simulink model "mypid2"  (R2024b)
settings: Solver=ode4  StartTime=0.0  StopTime=60  FixedStep=1e-3  RelTol=1e-3
StopFcn:
  | data = out.simout;
  | 
  | figure
  | subplot(2,1,1)
  | hold on
  | plot(data(:,1), data(:,2), 'LineWidth', 2, 'Color', 'r')
  | plot(data(:,1), data(:,3), 'LineWidth', 8, 'Color', 'b')
  | plot(data(:,1), data(:,4), 'LineWidth', 2, 'Color', 'k')
  | 
  | legend('Set vale', 'By MATLAB Simulink', 'By our discretization')
  | xlabel('Time (seconds)')
  | ylabel('Output')
  | 
  | subplot(2,1,2)
  | plot(data(:,1),abs(data(:,3)-data(:,4)), 'LineWidth', 2, 'Color', 'r')
  | xlabel('Time (seconds)')
  | ylabel('Absolute differences')
libraries: slpidlib x1, SignalEditorBlockLib x1
settings Model: Creator=auralius  LastModifiedBy=auralius

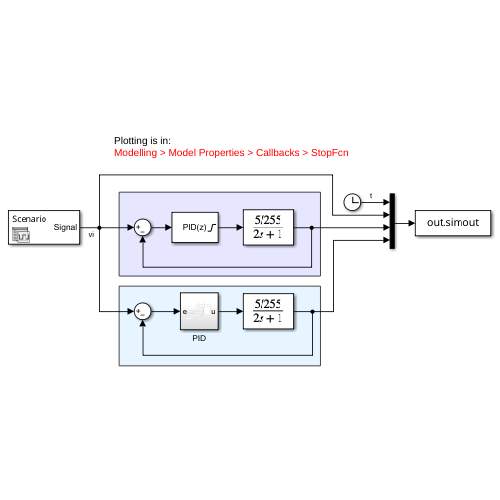
[thumbnail: Simulink's stored preview of the top-level diagram]
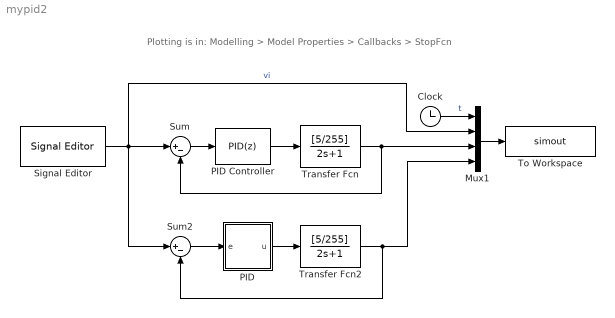
== system mypid2 ==
  note: Plotting is in:
      | Modelling > Model Properties > Callbacks > StopFcn
  Clock : Clock
  Mux1 : Mux
  PID : Subsystem
  PID Controller : slpidlib/PID Controller  Controller=PID  Form=Parallel  TimeDomain=Discrete-time  UseExternalTs=off  SampleTime=-1  IntegratorMethod=Trapezoidal  FilterMethod=Trapezoidal  ControllerParametersSource=internal  P=100  I=100  UseKiTs=off  D=10  UseExternalDerivativeSource=off  N=100  UseFilter=on  TunerSelectOption=Transfer Function Based (PID Tuner App)  ZeroCross=off  InitialConditionSource=internal  InitialConditionForIntegrator=0  InitialConditionForFilter=0  DifferentiatorICPrevScaledInput=0  ExternalReset=none  TrackingMode=off  Kt=1  LimitOutput=on  SatLimitsSource=internal  UpperSaturationLimit=255  LowerSaturationLimit=0  LinearizeAsGain=on  AntiWindupMode=clamping  Kb=1  LimitIntegrator=off  UpperIntegratorSaturationLimit=inf  LowerIntegratorSaturationLimit=-inf  POutMin=[]  POutMax=[]  IOutMin=[]  IOutMax=[]  DOutMin=[]  DOutMax=[]  NOutMin=[]  NOutMax=[]  SumOutMin=[]  SumOutMax=[]  SaturationOutDataTypeStr=Inherit: Inherit via back propagation  SaturationOutMin=[]  SaturationOutMax=[]  PParamMin=[]  PParamMax=[]  IParamMin=[]  IParamMax=[]  DParamMin=[]  DParamMax=[]  NParamMin=[]  NParamMax=[]  KbParamMin=[]  KbParamMax=[]  KtParamMin=[]  KtParamMax=[]  KbOutMin=[]  KbOutMax=[]  KtOutMin=[]  KtOutMax=[]  IntegratorOutMin=[]  IntegratorOutMax=[]  FilterOutMin=[]  FilterOutMax=[]  SumI1OutMin=[]  SumI1OutMax=[]  SumI2OutMin=[]  SumI2OutMax=[]  SumI3OutMin=[]  SumI3OutMax=[]  SumI4OutMin=[]  SumI4OutMax=[]  SumDOutMin=[]  SumDOutMax=[]  DifferentiatorOutMin=[]  DifferentiatorOutMax=[]  FilterDiffOutCoefMin=[]  FilterDiffOutCoefMax=[]  ReciprocalOutMin=[]  ReciprocalOutMax=[]  SumDenOutMin=[]  SumDenOutMax=[]  SumNumOutMin=[]  SumNumOutMax=[]  DivideOutMin=[]  DivideOutMax=[]  UdiffTsProdOutMin=[]  UdiffTsProdOutMax=[]  NTsProdOutMin=[]  NTsProdOutMax=[]  UintegralTsProdOutMin=[]  UintegralTsProdOutMax=[]  UngainTsProdOutMin=[]  UngainTsProdOutMax=[]  ClampingZeroOutDataTypeStr=Inherit: Inherit via back propagation  ClampingZeroOutMin=[]  ClampingZeroOutMax=[]  FilterDenConstantOutDataTypeStr=Inherit: Inherit via back propagation  FilterDenConstantOutMin=[]  FilterDenConstantOutMax=[]  PCopyOutDataTypeStr=Inherit: Inherit via back propagation  PCopyOutMin=[]  PCopyOutMax=[]  NCopyOutDataTypeStr=Inherit: Inherit via back propagation  NCopyOutMin=[]  NCopyOutMax=[]  IntegratorContinuousStateAttributes=''  IntegratorStateMustResolveToSignalObject=off  IntegratorRTWStateStorageClass=Auto  FilterContinuousStateAttributes=''  FilterStateMustResolveToSignalObject=off  FilterRTWStateStorageClass=Auto  ParallelPVariant=InternalParameters  IdealPVariant=Disabled  IVariant=InternalParameters  DVariant=InternalParameters  IntegratorVariant=Discrete  SatVariant=Enabled  AWVariant=DiscClampingParallel  PCopyVariant=Disabled  TRVariant=Disabled  FdbkBlocksVariant=Feedback  IdealPFdbkVariant=Passthrough  SatFdbkVariant=Passthrough  DerivativeFilterVariant=TrapezoidalFilter  NVariant=InternalParameters  NCopyVariant=InternalParameters  FilterICVariant=InternalICsFilter  IntegratorICVariant=InternalICs  ExternalResetVariant=Disabled  TRSumVariant=Passthrough  SumFdbkVariant=Enabled  SumVariant=Sum_PID  TsampFilterVariant=InternalTs  TsampNgainVariant=Passthrough  TsampIntegralVariant=Disabled_SignalSpec  ExternalSaturationOutDataTypeStr=Inherit: Same as second input  DerivativeSourceVariant=ErrorSignal  PreIntVariant=InternalPreInt
  Signal Editor : SignalEditorBlockLib/Signal Editor  FileName=test_signal.mat  ActiveScenario=Scenario  ActiveSignal=Signal  IsBus=off  OutputBusObjectStr=Bus: BusObject  SampleTime=0  Interpolate=off  ZeroCross=off  OutputAfterFinalValue=Setting to zero  Unit=inherit  PreserveSignalName=on  ApplySigPropsToAllScenarios=on  ApplySigPropsToAllSignals=off
  Sum : Sum  Inputs=|+-
  Sum2 : Sum  Inputs=|+-
  To Workspace : ToWorkspace  VariableName=simout  SampleTime=-1
      settings: Save2DSignal=2-D array (concatenate along first dimension)
  Transfer Fcn : TransferFcn  Numerator=[5/255]  Denominator=[2 1]
  Transfer Fcn2 : TransferFcn  Numerator=[5/255]  Denominator=[2 1]
  wires:
  Sum/1 -> PID Controller/1
  PID Controller/1 -> Transfer Fcn/1
  Transfer Fcn/1 -> Mux1/3, Sum/2
  Transfer Fcn2/1 -> Mux1/4, Sum2/2
  PID/1(u) -> Transfer Fcn2/1
  Sum2/1 -> PID/1(e)
  Clock/1 -> Mux1/1  "t"
  Signal Editor/1 -> Sum2/1, Sum/1, Mux1/2  "vi"
  Mux1/1 -> To Workspace/1

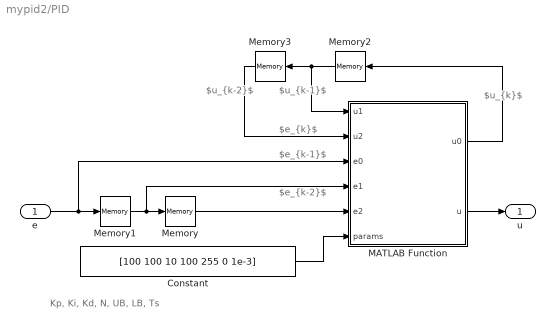
== system mypid2/PID ==
  note: Kp, Ki, Kd, N, UB, LB, Ts
  note: $u_{k-1}$
  note: $u_{k-2}$
  note: $u_{k}$
  note: $e_{k}$
  note: $e_{k-1}$
  note: $e_{k-2}$
  e : Inport
  Constant : Constant  Value=[100 100 10 100 255 0 1e-3]
  MATLAB Function : MATLAB Function  TreatAsAtomicUnit=on
  Memory{,1..3} (4 alike) : Memory  InheritSampleTime=on
  u : Outport
  wires:
  Memory3/1 -> MATLAB Function/2(u2)
  Memory/1 -> MATLAB Function/5(e2)
  Memory2/1 -> MATLAB Function/1(u1), Memory3/1
  Memory1/1 -> MATLAB Function/4(e1), Memory/1
  e/1 -> MATLAB Function/3(e0), Memory1/1
  MATLAB Function/2(u) -> u/1
  MATLAB Function/1(u0) -> Memory2/1
  Constant/1 -> MATLAB Function/6(params)

== matlab function mypid2/PID/MATLAB Function ==
  data: u0 output; u1 input; u2 input; e0 input; u output; e1 input; e2 input; params input
function [u0, u] = PID(u1, u2, e0, e1, e2, params)
% u1 is u(k-1)
% u2 is u(k-2)
% e0 is e(k)
% e1 is e(k-1)
% e2 is e(k-2)

Kp = params(1);
Ki = params(2);  
Kd = params(3); 
N  = params(4); 
UB = params(5); % lower-bound value for the saturated output
LB = params(6); % upper-bound value for the saturated output

Ts  = params(7);
NTs = N * Ts;

% PID
E0 = Kd/(2*Ts) + Ki*Ts/8 + Ki/(4*N) + Kp/4 + Kp/(2*NTs);
E1 = -Kd/Ts + Ki*Ts/4 - Kp/NTs;
E2 = Kd/(2*Ts) + Ki*Ts/8 - Ki/(4*N) - Kp/4 + Kp/(2*NTs);
lhs = (-1/NTs) * u1 + (-1/4 + 1/(2*NTs))*u2;
rhs = E0 * e0 + E1 * e1 + E2 * e2;
u_pid = (rhs - lhs) / (1/4 + 1/(2*NTs));

% With disabled integrator, Ki = 0
E0 = Kd/(2*Ts) + Kp/4 + Kp/(2*NTs);
E1 = -Kd/Ts - Kp/NTs;
E2 = Kd/(2*Ts) - Kp/4 + Kp/(2*NTs);
lhs = (-1/NTs) * u1 + (-1/4 + 1/(2*NTs))*u2;
rhs = E0 * e0 + E1 * e1 + E2 * e2;
u_pd = (rhs - lhs) / (1/4 + 1/(2*NTs));

if u_pid > UB
    u  = UB;
    u0 = u_pd;
elseif u_pid < LB
    u  = LB;
    u0 = u_pd;
else
    u  = u_pid;
    u0 = u_pid;
end
